simulink model "unprotected_left_turn_scenario1"  (R2020b)
settings: Solver=ode45  StartTime=0.0  StopTime=6  RelTol=1e-3
InitFcn:
  | global mdl;
  | mdl = run_setup_scenario1;
settings Model: Creator=swsmth  LastModifiedBy=swsmth
settings SolverCC: AlgebraicLoopSolver=LineSearch

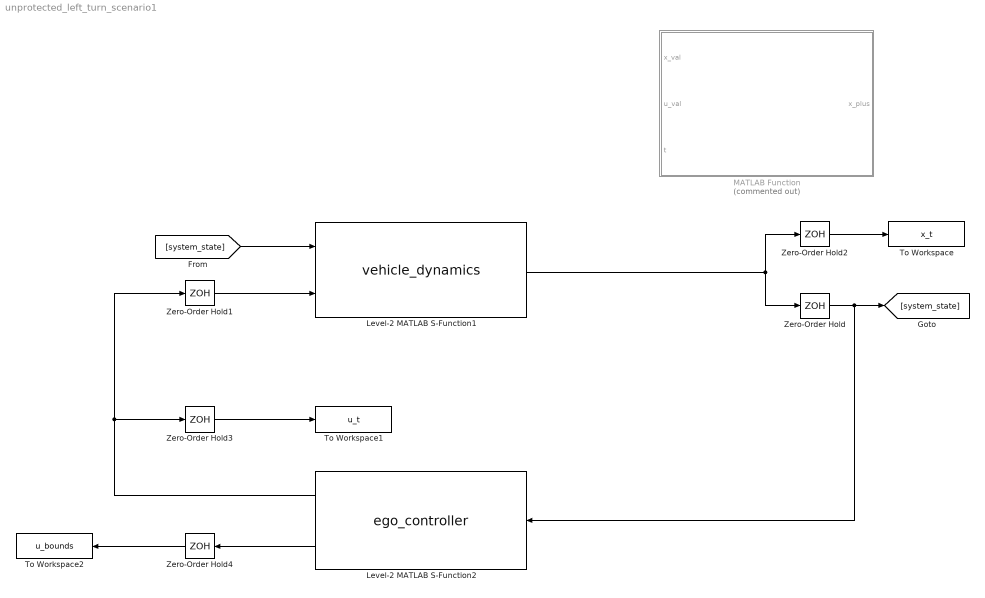
== system unprotected_left_turn_scenario1 ==
  Level-2 MATLAB S-Function1 : M-S-Function  FunctionName=vehicle_dynamics
  Level-2 MATLAB S-Function2 : M-S-Function  FunctionName=ego_controller
  MATLAB Function : MATLAB Function  Commented=on  TreatAsAtomicUnit=on
  To Workspace : ToWorkspace  VariableName=x_t  SampleTime=-1
  To Workspace1 : ToWorkspace  VariableName=u_t  SampleTime=-1
  To Workspace2 : ToWorkspace  VariableName=u_bounds  SampleTime=-1
  Zero-Order Hold : ZeroOrderHold  SampleTime=0.5
  Zero-Order Hold1 : ZeroOrderHold  SampleTime=0.01
  Zero-Order Hold2 : ZeroOrderHold  SampleTime=0.1
  Zero-Order Hold3 : ZeroOrderHold  SampleTime=0.1
  Zero-Order Hold4 : ZeroOrderHold  SampleTime=0.1
  wires:
  Zero-Order Hold2/1 -> To Workspace/1
  Zero-Order Hold3/1 -> To Workspace1/1
  Level-2 MATLAB S-Function2/2 -> Zero-Order Hold4/1
  Zero-Order Hold4/1 -> To Workspace2/1
  Zero-Order Hold/1 -> Level-2 MATLAB S-Function2/1, [system_state]
  Level-2 MATLAB S-Function1/1 -> Zero-Order Hold/1, Zero-Order Hold2/1
  [system_state] -> Level-2 MATLAB S-Function1/1
  Level-2 MATLAB S-Function2/1 -> Zero-Order Hold1/1, Zero-Order Hold3/1
  Zero-Order Hold1/1 -> Level-2 MATLAB S-Function1/2

== matlab function unprotected_left_turn_scenario1/MATLAB Function ==
  data: x_val input; x_plus output; u_val input; t input
function x_plus = vehicle_dynamics(x_val, u_val, t)

% TODO: make this nicer later!
%       (should be a way to read in parameters from global mdl variable)

% these values come from run_setup_scenario1.m

% set simulation parameters
mdl.x0 = [-42; 10.5; 0; -70];
mdl.v0 = 12;
mdl.v_min = 0;
mdl.v_max = 12;
mdl.v0_min = 8;
mdl.v0_max = 12;

% choose the parameters for our vehicle dynamics model
mdl.M = 2125;
mdl.R_w = 0.325;
mdl.alpha = 325;
mdl.beta = 0.175;
mdl.gamma = 0.475;

% sampling time
mdl.dt = 0.5;     % (for abstraction computations)
mdl.dt_sim = 0.1; % (for vehicle dynamics block in simulation)

if(t < 0.05)
    x_plus = mdl.x0;
else
    % from the modelling parameters, compute a, b, and c for each vehicle,
    % where we represent the dynamics for each vehicle as follows:
    %
    % \dot{p} = v,
    % \dot{v} = a + b * v + c * v^2,
    %
    % using our model, we have:
    %
    % a = (1 / con.M) * (T / con.R_w - con.alpha)
    %
    % b = - (1 / con.M) * con.beta
    %
    % c = - (1 / con.M) * con.gamma
    a = (1 / mdl.M) * (u_val / mdl.R_w - mdl.alpha);
    b = - (1 / mdl.M) * mdl.beta;
    c = - (1 / mdl.M) * mdl.gamma;
    
    % using numerical solution to vehicle dynamics eqn, compute next state
    x_plus = zeros(4, 1);
    [x_plus(1), x_plus(2)] = veh_dyn(x_val(1), x_val(2), a, b, c, mdl.dt_sim);
    x_plus(3) = x_val(3) + mdl.v0_min * mdl.dt_sim;
    x_plus(4) = x_val(4) + mdl.v0_max * mdl.dt_sim;
    
    % do thresholding on the ego vehicle velocity
    % (this is necessary because sometimes the ode45 solver lets
    % the ego vehicle go slightly outside of its velocity bounds)
    x_plus(2) = min(max(x_plus(2), mdl.v_min), mdl.v_max);
end

end

% compute next state
function [pos_plus, vel_plus] = veh_dyn(p0, v0, a, b, c, dt)
    
    % use ode45 solver to get state at next time step
    [t, x] = ode45(@f, [0 dt], [p0; v0; a; b; c]);
    
    % make sure we computed the state up until the sample time
    threshold = 1e-5;
    assert(abs(dt - t(end)) < threshold);
    
    % extract the position and velocity at time t = dt
    pos_plus = x(end, 1);
    vel_plus = x(end, 2);
    
end

function dxdt = f(t, x)

    % state convention is as follows:
    % x(1) = position,
    % x(2) = velocity,
    % x(3) = a,
    % x(4) = b,
    % x(5) = c
    
    % equations of motion, with state defined as above:
    dxdt = [x(2);
            x(3) + x(4) * x(2) + x(5) * x(2)^2;
            0;
            0;
            0];
    
    % ensure the vehicle does not reverse
    if(x(2) <= 0 && dxdt(2) < 0)
        dxdt(2) = 0;
    end
    
    % ensure the vehicle does not exceed its maximum velocity
    if(x(2) >= 12 && dxdt(2) > 0)
        dxdt(2) = 0;
    end
    
end
